simulink model "ActiveSuspension"  (R2024b)
settings: Solver=ode45  StartTime=0.0  StopTime=30  MaxStep=1e-4  RelTol=1e-3
values from neighbouring files (symbols this model uses):
  A = [  0,        1,         0,         0 ... (first row only)    [LQG.m]    (also in Poleproject.m = [0 0 1 0; changed.m; montecarlo.m; project3.m)
  B = [0 ... (first row only)    [LQG.m]    (also in Poleproject.m = [0 0; changed.m; montecarlo.m = [0; 1/mb; 0; -1/mw]; project3.m)
  K = place(A, Bf, desired_poles)    [Poleproject.m]    (also in changed.m = place(A, B, desired_poles); montecarlo.m = place(A, B, desired_poles); project3.m = place(A, B, desired_poles))
undefined symbols (not defined in the file or in its folder): B_obsv
libraries: simulink x1
settings Model: Creator=john_  LastModifiedBy=rakshitatelrandhe

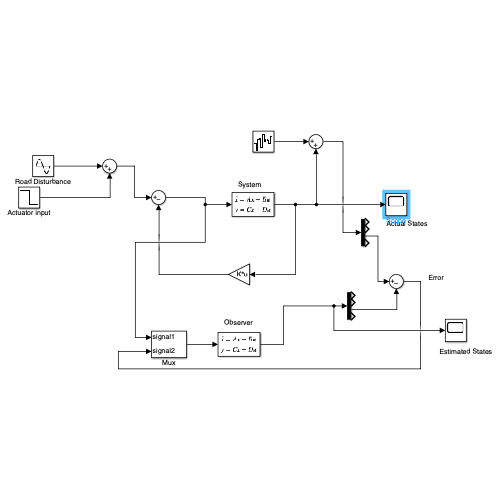
[thumbnail: Simulink's stored preview of the top-level diagram]
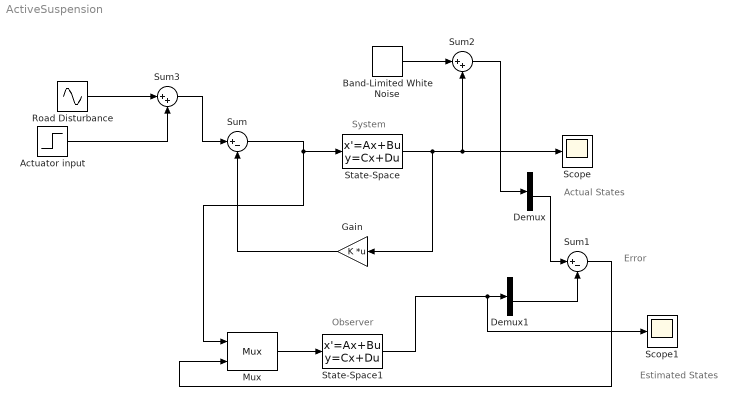
== system ActiveSuspension ==
  note: Observer
  note: System
  note: Error
  note: Actual States
  note: Estimated States
  Actuator input : Step  Before=10000  SampleTime=0
  Band-Limited White Noise : simulink/Sources/Band-Limited White Noise  Cov=0  Ts=0.1  seed=[23341]
  Demux : Demux
  Demux1 : Demux
  Gain : Gain  Gain=K  Multiplication=Matrix(K*u)
  Mux : Mux  Inputs=2
      settings: DisplayOption=signals
  Road Disturbance : Sin  Amplitude=500  SampleTime=0
  Scope : Scope
  Scope1 : Scope
  State-Space : StateSpace  A=A  B=B  C=[1 0 0 0; 0 1 0 0; 0 0 1 0; 0 0 0 1];  D=[0; 0; 0; 0]  InitialCondition=[0; 0; 0; 0]
  State-Space1 : StateSpace  A=A;  B=B_obsv;  C=[1 0 0 0; 0 1 0 0; 0 0 1 0; 0 0 0 1];  D=[0 0 0; 0 0 0; 0 0 0; 0 0 0];  InitialCondition=[0; 0; 0; 0];
  Sum : Sum  Inputs=|+-
  Sum1 : Sum  Inputs=|+-
  Sum2 : Sum  Inputs=|++
  Sum3 : Sum  Inputs=|++
  wires:
  Gain/1 -> Sum/2
  Sum/1 -> Mux/1, State-Space/1
  Mux/1 -> State-Space1/1
  Demux/3 -> Sum1/1
  Demux1/3 -> Sum1/2
  State-Space1/1 -> Scope1/1, Demux1/1
  Sum1/1 -> Mux/2
  Band-Limited White Noise/1 -> Sum2/1
  Sum2/1 -> Demux/1
  State-Space/1 -> Gain/1, Scope/1, Sum2/2
  Actuator input/1 -> Sum3/2
  Road Disturbance/1 -> Sum3/1
  Sum3/1 -> Sum/1
